simulink library "ComputeNorm3D"  (R2014b)
settings: Solver=ode45  StartTime=0.0  StopTime=10.0  RelTol=1e-3
settings Model: Creator=Hp  LastModifiedBy=Hp

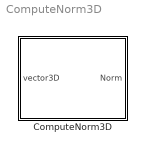
== system ComputeNorm3D ==
  ComputeNorm3D : Subsystem

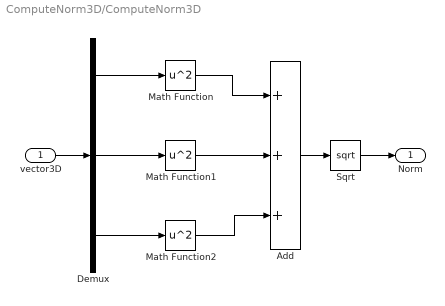
== system ComputeNorm3D/ComputeNorm3D ==
  vector3D : Inport
  Add : Sum  Inputs=+++
  Demux : Demux  Outputs=3
  Math Function : Math  Operator=square  SaturateOnIntegerOverflow=on
  Math Function1 : Math  Operator=square  SaturateOnIntegerOverflow=on
  Math Function2 : Math  Operator=square  SaturateOnIntegerOverflow=on
  Sqrt : Sqrt  SaturateOnIntegerOverflow=on
  Norm : Outport
  wires:
  Demux/2 -> Math Function1/1
  Demux/3 -> Math Function2/1
  Math Function/1 -> Add/1
  Demux/1 -> Math Function/1
  Math Function2/1 -> Add/3
  Math Function1/1 -> Add/2
  Add/1 -> Sqrt/1
  Sqrt/1 -> Norm/1
  vector3D/1 -> Demux/1
